simulink model "PIDtrueTime"  (R2019a)
settings: Solver=VariableStepAuto  StartTime=0.0  StopTime=40  RelTol=1e-3
libraries: cstblocks x1, truetime x1
settings Model: Creator=Alvaro UAO  LastModifiedBy=Alvaro UAO

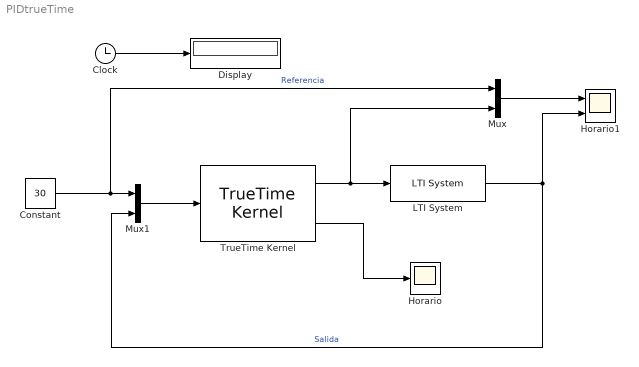
== system PIDtrueTime ==
  Clock : Clock
  Constant : Constant  Value=30
  Display : Display
      settings: Decimation=2
  Horario : Scope
  Horario1 : Scope  NumInputPorts=2
  LTI System : cstblocks/LTI System  sys=PlantaTot  IC=[]
  Mux : Mux  Inputs=2
  Mux1 : Mux  Inputs=2
  TrueTime Kernel : truetime/TrueTime Kernel  sfun=initPID  args=4  ninputsoutputs=[2 1]  ntriggers=0  trigtype=falling  nwnodenbr=[]  clockoffsetdrift=[0 0]  schedoutput=on  battery=off  poweroutput=off
  wires:
  TrueTime Kernel/1 -> Mux/2, LTI System/1
  TrueTime Kernel/2 -> Horario/1
  Mux/1 -> Horario1/1
  LTI System/1 -> Mux1/2, Horario1/2  "Salida"
  Mux1/1 -> TrueTime Kernel/1
  Constant/1 -> Mux/1, Mux1/1  "Referencia"
  Clock/1 -> Display/1
